simulink model "internal_loop"  (R2025b)
settings: Solver=ode45  StartTime=0.0  StopTime=sim_stop_time  MaxStep=sim_step_time  RelTol=1e-8  AbsTol=1e-8
undefined symbols (not defined in the file): B_total, C2RAD_TS_gain, DCB2V, Jm, K, kd, ki, kp, Lgain, Lm, RAD2C_gain, ref_speed, Rm, sat_limit, sim_step_time, TS, V2DCB, vref
libraries: simulink x1, slpidlib x1
settings Model: Creator=shashi  LastModifiedBy=shashi
settings SolverCC: AutoScaleAbsTol=off
settings DataIOCC: SaveOutput=off  SignalLogging=off  DSMLogging=off  SaveTime=off  ReturnWorkspaceOutputs=off

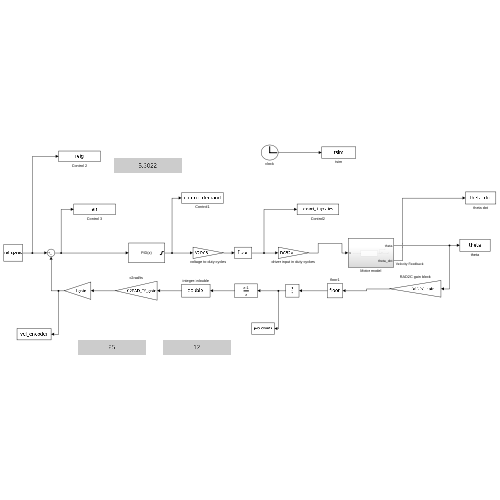
[thumbnail: Simulink's stored preview of the top-level diagram]
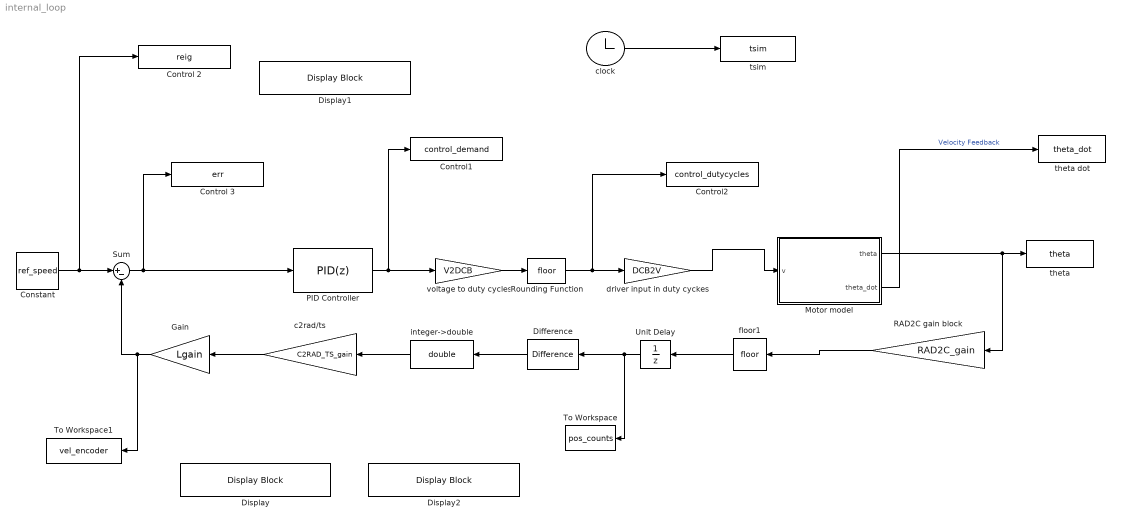
== system internal_loop ==
  Constant : Constant  Value=ref_speed  SampleTime=sim_step_time
  Control 2 : ToWorkspace  VariableName=reig  SampleTime=sim_step_time
      settings: Save2DSignal=2-D array (concatenate along first dimension)
  Control 3 : ToWorkspace  VariableName=err  SampleTime=sim_step_time
      settings: Save2DSignal=2-D array (concatenate along first dimension)
  Control1 : ToWorkspace  VariableName=control_demand  SampleTime=sim_step_time
      settings: Save2DSignal=2-D array (concatenate along first dimension)
  Control2 : ToWorkspace  VariableName=control_dutycycles  SampleTime=sim_step_time
      settings: Save2DSignal=2-D array (concatenate along first dimension)
  Difference : simulink/Discrete/Difference  ICPrevInput=0.0  OutMin=[]  OutMax=[]  OutDataType=fixdt(1, 16)  OutScaling=2^-10  DoSatur=off
  Display : DisplayBlock  LabelPosition=Hide  Transparency=1  GridColor=[0.502, 0.502, 0.502]
  Display1 : DisplayBlock  LabelPosition=Hide  Transparency=1  GridColor=[0.502, 0.502, 0.502]
  Display2 : DisplayBlock  LabelPosition=Hide  Transparency=1  GridColor=[0.502, 0.502, 0.502]
  Gain : Gain  Gain=Lgain
  Motor model : Subsystem
  PID Controller : slpidlib/PID Controller  Controller=PID  Form=Parallel  TimeDomain=Discrete-time  UseExternalTs=off  SampleTime=TS  IntegratorMethod=Forward Euler  FilterMethod=Forward Euler  ControllerParametersSource=internal  P=kp  I=ki  UseKiTs=off  D=kd  UseExternalDerivativeSource=off  N=100  UseFilter=on  TunerSelectOption=Transfer Function Based (PID Tuner App)  InitialConditionSource=internal  InitialConditionForIntegrator=0  InitialConditionForFilter=0  DifferentiatorICPrevScaledInput=0  ExternalReset=none  TrackingMode=off  Kt=1  LimitOutput=on  SatLimitsSource=internal  UpperSaturationLimit=sat_limit  LowerSaturationLimit=-sat_limit  LinearizeAsGain=on  AntiWindupMode=back-calculation  Kb=1  LimitIntegrator=off  UpperIntegratorSaturationLimit=vref  LowerIntegratorSaturationLimit=-vref  POutMin=[]  POutMax=[]  IOutMin=[]  IOutMax=[]  DOutMin=[]  DOutMax=[]  NOutMin=[]  NOutMax=[]  SumOutMin=[]  SumOutMax=[]  SaturationOutMin=[]  SaturationOutMax=[]  PParamMin=[]  PParamMax=[]  IParamMin=[]  IParamMax=[]  DParamMin=[]  DParamMax=[]  NParamMin=[]  NParamMax=[]  KbParamMin=[]  KbParamMax=[]  KtParamMin=[]  KtParamMax=[]  KbOutMin=[]  KbOutMax=[]  KtOutMin=[]  KtOutMax=[]  IntegratorOutMin=[]  IntegratorOutMax=[]  FilterOutMin=[]  FilterOutMax=[]  SumI1OutMin=[]  SumI1OutMax=[]  SumI2OutMin=[]  SumI2OutMax=[]  SumI3OutMin=[]  SumI3OutMax=[]  SumI4OutMin=[]  SumI4OutMax=[]  SumDOutMin=[]  SumDOutMax=[]  DifferentiatorOutMin=[]  DifferentiatorOutMax=[]  FilterDiffOutCoefMin=[]  FilterDiffOutCoefMax=[]  ReciprocalOutMin=[]  ReciprocalOutMax=[]  SumDenOutMin=[]  SumDenOutMax=[]  SumNumOutMin=[]  SumNumOutMax=[]  DivideOutMin=[]  DivideOutMax=[]  UdiffTsProdOutMin=[]  UdiffTsProdOutMax=[]  NTsProdOutMin=[]  NTsProdOutMax=[]  UintegralTsProdOutMin=[]  UintegralTsProdOutMax=[]  UngainTsProdOutMin=[]  UngainTsProdOutMax=[]  ClampingZeroOutDataTypeStr=Inherit: Inherit via back propagation  ClampingZeroOutMin=[]  ClampingZeroOutMax=[]  FilterDenConstantOutDataTypeStr=Inherit: Inherit via back propagation  FilterDenConstantOutMin=[]  FilterDenConstantOutMax=[]  PCopyOutDataTypeStr=Inherit: Inherit via back propagation  PCopyOutMin=[]  PCopyOutMax=[]  NCopyOutDataTypeStr=Inherit: Inherit via back propagation  NCopyOutMin=[]  NCopyOutMax=[]  IntegratorContinuousStateAttributes=''  IntegratorStateMustResolveToSignalObject=off  IntegratorRTWStateStorageClass=Auto  FilterContinuousStateAttributes=''  FilterStateMustResolveToSignalObject=off  FilterRTWStateStorageClass=Auto  ParallelPVariant=InternalParameters  IdealPVariant=Disabled  IVariant=InternalParameters  DVariant=InternalParameters  IntegratorVariant=Discrete  SatVariant=Enabled  AWVariant=BackCalculation  PCopyVariant=Disabled  TRVariant=Disabled  FdbkBlocksVariant=Forward  IdealPFdbkVariant=Disabled  SatFdbkVariant=Disabled  DerivativeFilterVariant=ForwardEulerFilter  NVariant=InternalParameters  NCopyVariant=Disabled  FilterICVariant=InternalICsFilter  IntegratorICVariant=InternalICs  ExternalResetVariant=Disabled  TRSumVariant=Passthrough  SumFdbkVariant=Disabled  SumVariant=Sum_PID  TsampFilterVariant=InternalTs  TsampNgainVariant=Passthrough  TsampIntegralVariant=Disabled_SignalSpec  ExternalSaturationOutDataTypeStr=Inherit: Same as second input  DerivativeSourceVariant=ErrorSignal  PreIntVariant=InternalPreInt
  RAD2C gain block : Gain  Gain=RAD2C_gain
  Rounding Function : Rounding
  Sum : Sum  Inputs=|+-
  To Workspace : ToWorkspace  VariableName=pos_counts  SampleTime=TS
      settings: Save2DSignal=2-D array (concatenate along first dimension)
  To Workspace1 : ToWorkspace  VariableName=vel_encoder  SampleTime=TS
      settings: Save2DSignal=2-D array (concatenate along first dimension)
  Unit Delay : UnitDelay  SampleTime=TS  HasFrameUpgradeWarning=on
  c2rad/ts : Gain  Gain=C2RAD_TS_gain
  clock : Clock
  driver input in duty cyckes : Gain  Gain=DCB2V
  floor1 : Rounding
  integer->double : DataTypeConversion  OutDataTypeStr=double  SaturateOnIntegerOverflow=off  RndMeth=Floor
  theta : ToWorkspace  VariableName=theta  SampleTime=sim_step_time
      settings: Save2DSignal=2-D array (concatenate along first dimension)
  theta dot : ToWorkspace  VariableName=theta_dot  SampleTime=sim_step_time
      settings: Save2DSignal=2-D array (concatenate along first dimension)
  tsim : ToWorkspace  VariableName=tsim  SampleTime=sim_step_time
      settings: Save2DSignal=2-D array (concatenate along first dimension)
  voltage to duty cycles : Gain  Gain=V2DCB
  wires:
  clock/1 -> tsim/1
  Constant/1 -> Sum/1, Control 2/1
  Motor model/1(theta) -> RAD2C gain block/1, theta/1
  Motor model/2(theta_dot) -> theta dot/1  "Velocity Feedback"
  Sum/1 -> Control 3/1, PID Controller/1
  PID Controller/1 -> voltage to duty cycles/1, Control1/1
  voltage to duty cycles/1 -> Rounding Function/1
  Rounding Function/1 -> driver input in duty cyckes/1, Control2/1
  RAD2C gain block/1 -> floor1/1
  floor1/1 -> Unit Delay/1
  Unit Delay/1 -> To Workspace/1, Difference/1
  Difference/1 -> integer->double/1
  integer->double/1 -> c2rad/ts/1
  c2rad/ts/1 -> Gain/1
  Gain/1 -> To Workspace1/1, Sum/2
  driver input in duty cyckes/1 -> Motor model/1(v)

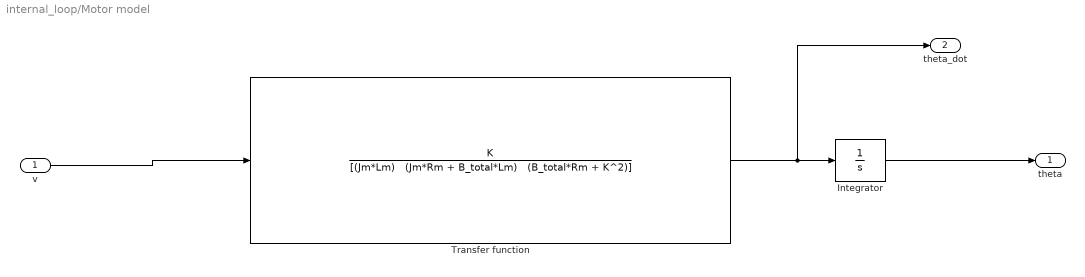
== system internal_loop/Motor model ==
  v : Inport
  Integrator : Integrator
  Transfer function : TransferFcn  Numerator=K  Denominator="[(Jm*Lm)   (Jm*Rm + B_total*Lm)   (B_total*Rm + K^2)]"
  theta : Outport
  theta_dot : Outport  Port=2
  wires:
  v/1 -> Transfer function/1
  Transfer function/1 -> theta_dot/1, Integrator/1
  Integrator/1 -> theta/1
